simulink library "Kind"  (R2017a)
settings: Solver=VariableStepAuto  StartTime=0.0  StopTime=10.0  RelTol=1e-3
settings Model: Creator=mudat  LastModifiedBy=mudat

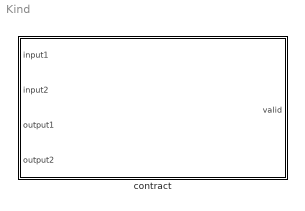
== system Kind ==
  contract : Subsystem

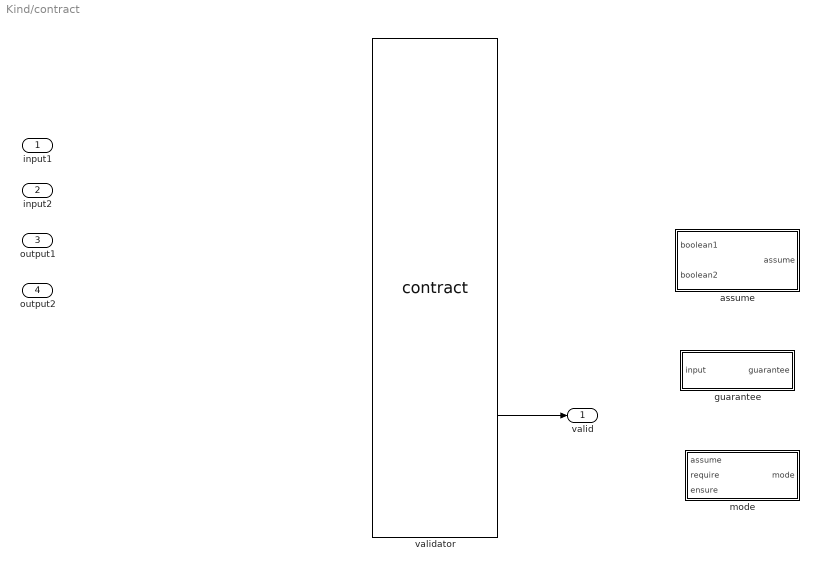
== system Kind/contract ==
  input1 : Inport
  input2 : Inport  Port=2
  output1 : Inport  Port=3
  output2 : Inport  Port=4
  assume : Subsystem
  guarantee : Subsystem
  mode : Subsystem
  validator : M-S-Function  FunctionName=contract  mask{assumePorts=2, guaranteePorts=2, modePorts=2}
      mask prompts: assumePorts "Assume ports     :"; guaranteePorts "Guarantee ports :"; modePorts "Mode ports        :"
      mask init:
      | set_param(gcb,'LinkStatus','none');
      mask Callback modePorts: contract_callback('inputs_callback',gcb)
      mask Display:
      | port_label('input',1,'assume')
      | port_label('input',2,'assume')
      | port_label('input',3,'guarantee')
      | port_label('input',4,'guarantee')
      | port_label('input',5,'mode')
      | port_label('input',6,'mode')
      | port_label('output',1,'assume')
      | port_label('output',2,'valid')
  valid : Outport
  wires:
  validator/2 -> valid/1

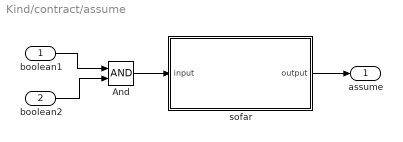
== system Kind/contract/assume ==
  boolean1 : Inport  OutDataTypeStr=boolean
  boolean2 : Inport  Port=2  OutDataTypeStr=boolean
  And : Logic  IconShape=distinctive  AllPortsSameDT=off  OutDataTypeStr=boolean
  sofar : Subsystem
  assume : Outport  OutDataTypeStr=boolean
  wires:
  boolean2/1 -> And/2
  boolean1/1 -> And/1
  And/1 -> sofar/1(input)
  sofar/1(output) -> assume/1

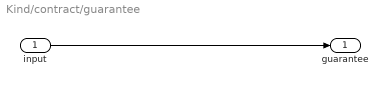
== system Kind/contract/guarantee ==
  input : Inport  OutDataTypeStr=boolean
  guarantee : Outport  OutDataTypeStr=boolean
  wires:
  input/1 -> guarantee/1

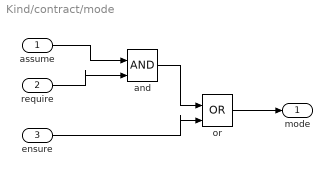
== system Kind/contract/mode ==
  assume : Inport  OutDataTypeStr=boolean
  require : Inport  Port=2  OutDataTypeStr=boolean
  ensure : Inport  Port=3  OutDataTypeStr=boolean
  and : Logic  IconShape=distinctive  AllPortsSameDT=off  OutDataTypeStr=boolean
  or : Logic  Operator=OR  IconShape=distinctive  AllPortsSameDT=off  OutDataTypeStr=boolean
  mode : Outport
  wires:
  assume/1 -> and/1
  require/1 -> and/2
  or/1 -> mode/1
  and/1 -> or/1
  ensure/1 -> or/2

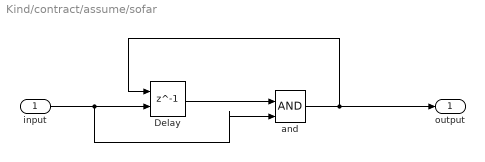
== system Kind/contract/assume/sofar ==
  input : Inport  OutDataTypeStr=boolean
  Delay : Delay  DelayLength=1  InitialConditionSource=Input port
      settings: InputPortMap=u0,p4
  and : Logic  IconShape=distinctive  AllPortsSameDT=off  OutDataTypeStr=boolean
  output : Outport
  wires:
  input/1 -> Delay/2, and/2
  Delay/1 -> and/1
  and/1 -> Delay/1, output/1
